simulink model "Week3_Problem3"  (R2020b)
settings: Solver=ode45  StartTime=0.0  StopTime=10.0  RelTol=1e-3
PreLoadFcn:
  | LookupTableVariables.m
PostLoadFcn:
  | posRef=[-10 0 0;-8.5000000389649344 -0.00032057688834367633 0;-7.00000013243916 0.0001046627707353404 0;-5.5000013719066843 0.0019633028915715441 0;-4.0000068200170222 0.0059429239765455251 0;-2.500022456114432 0.012731095719916501 0;-1.000058121729845 0.023015362926791384 0;0.49987153401052709 0.037483222580328462 0;1.9997488741214804 0.05661776191230368 0;3.4995533957878173 0.0807832726616669 0;4.9992537956041394 0.11070949504224792 0;6.4988102169399058 0.14713214905782759 0;7.99817323834591 0.19078661801418004 0;9.4972827923589911 0.24240782912164788 0;10.996067085850811 0.3027301079820538 0;12.494441522418191 0.37248700431913734 0;13.992307627411369 0.45241108632067739 0;15.489552329450575 0.54322828982636229 0;16.986104748171872 0.64482692871996372 0;18.481993555798578 0.75577957443767907 0;19.977281971545665 0.87455822436566311 0;21.472057156443615 0.99963648279861006 0;22.966425539696488 1.1294893996997795 0;24.46050815174387 1.2625932112379594 0;25.954435963048805 1.3974250059040985 0;27.448345227102681 1.5324623399719128 0;28.942364285176254 1.6662786950018476 0;30.43653068335416 1.7984397038989934 0;31.93085365809711 1.9288182087711181 0;33.425345542750946 2.0572458498503861 0;34.920018011779121 2.1835542137146304 0;36.414882023832668 2.3075748302864034 0;37.909947764790829 2.429139170234988 0;39.405224590771311 2.5480786428134428 0;40.900720971109862 2.6642245941628082 0;42.396444431308815 2.7774083061155972 0;43.892403246150053 2.8874369946783749 0;45.38861538488505 2.9939643927789104 0;46.885100476364542 3.096584841736945 0;48.381874979464556 3.1948924196190918 0;49.878951847726285 3.2884810058016432 0;51.37634019890595 3.3769442815837016 0;52.874044984321365 3.4598757359962891 0;54.372066658021069 3.5368686772556726 0;55.870400845812341 3.6075162503092817 0;57.369038014196278 3.671411460922684 0;58.8679627576989 3.7281578592117861 0;60.367140794768574 3.7777688127128712 0;61.866523659152122 3.8207531578250689 0;63.366068909506666 3.8576478218748256 0;64.865740653375155 3.88899000870342 0;66.3655089701928 3.9153171356111991 0;67.865349333770865 3.937166781005621 0;69.365242034387677 3.9550766417191987 0;70.865171600593058 3.9695844989622167 0;72.365126220810183 3.9812281918741537 0;73.865097164799934 3.9905455976371416 0;75.365078205036667 3.9980746171143191 0;76.86506555014661 4.0042226492204165 0;78.365058007335023 4.0089633882717308 0;79.86505400366265 4.0124108908590994 0;81.36505223070516 4.0146952649335228 0;82.8650516827077 4.0159466197411575 0;84.3650516227284 4.0162950653504659 0;85.865051548781452 4.01587071229594 0;87.365051159979728 4.01480367132374 0;88.865050322677291 4.013224053224536 0;90.365049036611751 4.0112619687388946 0;91.865047401046667 4.0090475285205036 0;93.365045580914 4.0067108431425709 0;94.865043772956454 4.0043820231326963 0;96.365042171870044 4.0021911790215441 0;97.865040936446476 4.0002684213906274 0;99.365040171863072 3.9987605666119856 0;100.86503980649982 3.9977214126735334 0;102.36503967169195 3.9970952314177151 0;103.86503964436331 3.9968249528974638 0;105.36503964206052 3.9968535071325086 0;106.86503961643893 3.9971238241271045 0;108.36503954674873 3.997578833881275 0;109.86503943332092 3.9981614663968053 0;111.36503929105332 3.9988146516792265 0;112.86503914289671 3.9994813197370265 0]
  | t= [0 0.099999999999999992 0.20000000000000004 0.3000000000000001 0.40000000000000019 0.50000000000000022 0.60000000000000031 0.7000000000000004 0.80000000000000049 0.90000000000000058 1.0000000000000007 1.1000000000000008 1.2000000000000008 1.3000000000000009 1.400000000000001 1.5000000000000011 1.6000000000000012 1.7000000000000013 1.8000000000000014 1.9000000000000015 2.0000000000000013 2.0999999999999992 2.1999999999999971 2.2999999999999949 2.3999999999999928 2.4999999999999907 2.5999999999999885 2.6999999999999864 2.7999999999999843 2.8999999999999821 2.99999999999998 3.0999999999999779 3.1999999999999758 3.2999999999999736 3.3999999999999715 3.4999999999999694 3.5999999999999672 3.6999999999999651 3.799999999999963 3.8999999999999608 3.9999999999999587 4.099999999999957 4.1999999999999549 4.2999999999999527 4.3999999999999506 4.4999999999999485 4.5999999999999464 4.6999999999999442 4.7999999999999421 4.89999999999994 4.9999999999999378 5.0999999999999357 5.1999999999999336 5.2999999999999314 5.3999999999999293 5.4999999999999272 5.599999999999925 5.6999999999999229 5.7999999999999208 5.8999999999999186 5.9999999999999165 6.0999999999999144 6.1999999999999122 6.29999999999991 6.399999999999908 6.4999999999999059 6.5999999999999037 6.6999999999999016 6.7999999999998995 6.8999999999998973 6.9999999999998952 7.0999999999998931 7.1999999999998909 7.2999999999998888 7.3999999999998867 7.4999999999998845 7.5999999999998824 7.69999999999988 7.7999999999998781 7.899999999999876 7.9999999999998739 8.0999999999998717 8.19999999999987]
  | yawRef = [-0.017734585131802181 -0.0023783867480744541 0.039241603596663142 0.10712538590241065 0.20127296016916807 0.32168432639693528 0.46835948458571258 0.64129843473549952 0.82243120441432782 1.0284466171618847 1.2625895772261897 1.5248600846072435 1.8152581393050453 2.133783741319597 2.4804368906508958 2.8552175872989438 3.2581258312637407 3.6852031921171342 4.0725918737692446 4.4015950546183911 4.6722127346645754 4.8844449139077941 5.0382915923480533 5.1337527699853531 5.1708284468196917 5.1495186228510716 5.0867585477276682 5.02163347038271 4.95006090740082 4.872040858781995 4.787573324526238 4.6966583046335471 4.5992957991039214 4.4954858079373627 4.3852283311338685 4.268523368693443 4.1421046794896679 4.00026229516887 3.8429080694151376 3.6700420022284757 3.4816640936088827 3.2777743435563571 3.058372752070901 2.823459319152513 2.5730340448011941 2.3070969290169434 2.0288148473761831 1.7653020474819436 1.522336655896058 1.2999186726185261 1.0980480976493481 0.91672493098852348 0.75594917263605244 0.61572082259193561 0.49603988085617257 0.39690634742876296 0.3183202223097073 0.26028150549900531 0.20743891230476702 0.155555799189824 0.10864254782766856 0.066699158218300636 0.029725630361720226 -0.0022780357420727169 -0.0293118400930781 -0.051375782691295953 -0.068469863536726308 -0.080594082629369151 -0.087748439969224434 -0.0899329355562922 -0.087147569390572471 -0.079392341472065239 -0.066667251800770516 -0.04830659623807302 -0.031442242528749914 -0.016757802096312908 -0.004253274940762026 0.0060713389379027606 0.014216039539681403 0.020180826864573963 0.023965700912580403 0.025570661683700712 0.024995709177934915]
model workspace (MAT data in the model file):
  mpc1 = mpc
  mpc1.Ts = 0.1
  mpc1.PredictionHorizon = 10
  mpc1.ControlHorizon = 3
  mpc1.Model.Plant = ss
  mpc1.Model.Plant.InputName_ = "Steering angle"
  mpc1.Model.Plant.InputUnit_ = "rad"
  mpc1.Model.Plant.InputGroup_.Manipulated = 1
  mpc1.Model.Plant.OutputName_ = ["Lateral position"; "Yaw angle"]
  mpc1.Model.Plant.OutputUnit_ = ["m"; "rad"]
  mpc1.Model.Plant.OutputGroup_.Measured = [1 2]
  mpc1.Model.Plant.IOSize_ = [2 1]
  mpc1.Model.Plant.Data_ = ltipack.ssdata
  mpc1.Model.Plant.Data_.StateName = ["Plant(1)"; "Plant(2)"; "Plant(3)"; "Plant(4)"]
  mpc1.Model.Plant.Data_.a = [0.590295220137  0  -0.749548819532  0; 0.00501866857034  1  0.0760340469864  0; 0.0836937369247  0  0.543093723808  0; 0.0815953844705  1.5  0.0178017333486  1]
  mpc1.Model.Plant.Data_.b = [1.18987189092; 0.0707419750471; 1.3270514387; 0.114007098227]
  mpc1.Model.Plant.Data_.c = [0  0  0  1; 0  1  0  0]
  mpc1.Model.Plant.Data_.d = [0; 0]
  mpc1.Model.Plant.Data_.Delay.Input = 0
  mpc1.Model.Plant.Data_.Delay.Output = [0; 0]
  mpc1.Model.Plant.Data_.Delay.Internal = []
  mpc1.Model.Plant.Data_.Ts = 0.1
  mpc1.Model.Disturbance = []
  mpc1.Model.Noise = []
  mpc1.Model.Nominal.X = [0; 0; 0; 0]
  mpc1.Model.Nominal.DX = [0; 0; 0; 0]
  mpc1.Model.Nominal.U = 0
  mpc1.Model.Nominal.Y = [0; 0]
  mpc1.ManipulatedVariables.Min = -0.523598775598
  mpc1.ManipulatedVariables.Max = 0.523598775598
  mpc1.ManipulatedVariables.MinECR = 0
  mpc1.ManipulatedVariables.MaxECR = 0
  mpc1.ManipulatedVariables.RateMin = -0.261799387799
  mpc1.ManipulatedVariables.RateMax = 0.261799387799
  mpc1.ManipulatedVariables.RateMinECR = 0
  mpc1.ManipulatedVariables.RateMaxECR = 0
  mpc1.ManipulatedVariables.Target = 'nominal'
  mpc1.ManipulatedVariables.Name = 'Steering angle'
  mpc1.ManipulatedVariables.Units = 'rad'
  mpc1.ManipulatedVariables.ScaleFactor = 1
  mpc1.OutputVariables(1).Min = -2
  mpc1.OutputVariables(1).Max = 6
  mpc1.OutputVariables(1).MinECR = 1
  mpc1.OutputVariables(1).MaxECR = 1
  mpc1.OutputVariables(1).Name = 'Lateral position'
  mpc1.OutputVariables(1).Units = 'm'
  mpc1.OutputVariables(1).ScaleFactor = 1
  mpc1.OutputVariables(2).Min = -0.2
  mpc1.OutputVariables(2).Max = 0.2
  mpc1.OutputVariables(2).MinECR = 1
  mpc1.OutputVariables(2).MaxECR = 1
  mpc1.OutputVariables(2).Name = 'Yaw angle'
  mpc1.OutputVariables(2).Units = 'rad'
  mpc1.OutputVariables(2).ScaleFactor = 1
  mpc1.Weights.ManipulatedVariables = 0
  mpc1.Weights.ManipulatedVariablesRate = 0.0353454681959
  mpc1.Weights.OutputVariables = [2.82921701435 0.282921701435]
  mpc1.Weights.ECR = 100000
  mpc1.Optimizer.Algorithm = 'active-set'
  mpc1.Optimizer.ActiveSetOptions.MaxIterations = 'default'
  mpc1.Optimizer.ActiveSetOptions.ConstraintTolerance = 1e-06
  mpc1.Optimizer.ActiveSetOptions.UseWarmStart = 1
  mpc1.Optimizer.InteriorPointOptions.MaxIterations = 50
  mpc1.Optimizer.InteriorPointOptions.ConstraintTolerance = 1e-06
  mpc1.Optimizer.InteriorPointOptions.OptimalityTolerance = 1e-06
  mpc1.Optimizer.InteriorPointOptions.ComplementarityTolerance = 1e-08
  mpc1.Optimizer.InteriorPointOptions.StepTolerance = 1e-08
  mpc1.Optimizer.MinOutputECR = 0
  mpc1.Optimizer.UseSuboptimalSolution = 0
  mpc1.Optimizer.CustomSolver = 0
  mpc1.Optimizer.CustomSolverCodeGen = 0
  mpc1.History = [2018 8 28 11 8 30.674]
  mpc1.MPCData = mpcdata
  mpc1.MPCData.IsDirty = 1
  mpc1.MPCData.Ts = 0.1
  mpc1.MPCData.p = 10
  mpc1.MPCData.m = 3
  mpc1.MPCData.UseActiveSetSolver = 1
  mpc1.MPCData.UseSuboptimalSolution = 0
  mpc1.MPCData.CustomSolver = 0
  mpc1.MPCData.CustomSolverCodeGen = 0
  mpc1.MPCData.IsCustomEstimation = 0
  mpc1.MPCData.Uscale = 1
  mpc1.MPCData.Yscale = [1; 1]
  mpc1.MPCData.mvindex = 1
  mpc1.MPCData.myindex = [1; 2]
  mpc1.IsEmpty = 0
  mpc1.OldOVIntegrator = {[]; []}
  mpc1.Version = '6.1'
  posRef = [-10 -8.50000003896 -7.00000013244 -5.50000137191 -4.00000682002 -2.50002245611 -1.00005812173 0.499871534011 1.99974887412 3.49955339579 4.9992537956 6.49881021694 ... (249 elements, 83x3)]
  t = [0 0.1 0.2 0.3 0.4 0.5 0.6 0.7 0.8 0.9 1 1.1 1.2 1.3 1.4 1.5 1.6 1.7 1.8 1.9 2 2.1 2.2 2.3 2.4 2.5 2.6 2.7 2.8 2.9 3 3.1 3.2 3.3 3.4 3.5 3.6 3.7 3.8 3.9 4 4.1 4.2 4.3 4.4 4.5 4.6 4.7 4.8 4.9 5 5.1 5.2 5.3 5.4 5.5 5.6 5.7 5.8 5.9 6 6.1 6.2 6.3 6.4 6.5 6.6 6.7 6.8 6.9 7 7.1 7.2 7.3 7.4 7.5 7.6 7.7 7.8 7.9 8 8.1 8.2]
  yawRef = [-0.0177345851318 -0.00237838674807 0.0392416035967 0.107125385902 0.201272960169 0.321684326397 0.468359484586 0.641298434735 0.822431204414 1.02844661716 1.26258957723 1.52486008461 1.81525813931 2.13378374132 2.48043689065 2.8552175873 3.25812583126 3.68520319212 4.07259187377 4.40159505462 4.67221273466 4.88444491391 5.03829159235 5.13375276999 5.17082844682 5.14951862285 5.08675854773 5.02163347038 4.9500609074 4.87204085878 4.78757332453 4.69665830463 4.5992957991 4.49548580794 4.38522833113 4.26852336869 4.14210467949 4.00026229517 3.84290806942 3.67004200223 3.48166409361 3.27777434356 3.05837275207 2.82345931915 2.5730340448 2.30709692902 2.02881484738 1.76530204748 1.5223366559 1.29991867262 1.09804809765 0.916724930989 0.755949172636 0.615720822592 0.496039880856 0.396906347429 0.31832022231 0.260281505499 0.207438912305 0.15555579919 0.108642547828 0.0666991582183 0.0297256303617 -0.00227803574207 -0.0293118400931 -0.0513757826913 -0.0684698635367 -0.0805940826294 -0.0877484399692 -0.0899329355563 -0.0871475693906 -0.0793923414721 -0.0666672518008 -0.0483065962381 -0.0314422425287 -0.0167578020963 -0.00425327494076 0.0060713389379 0.0142160395397 0.0201808268646 0.0239657009126 0.0255706616837 0.0249957091779]
values from neighbouring files (symbols this model uses):
  desiredLong = [20 24 30]    [LookupTableVariables.m]
  givenLong = [ 10 12 15]    [LookupTableVariables.m]
undefined symbols (not defined in the file or in its folder): sigbuilder_block
libraries: mpclib x1
CloseFcn:
  | clearvars
settings Model: OrderedModelArguments=off  Creator=hp  LastModifiedBy=hp

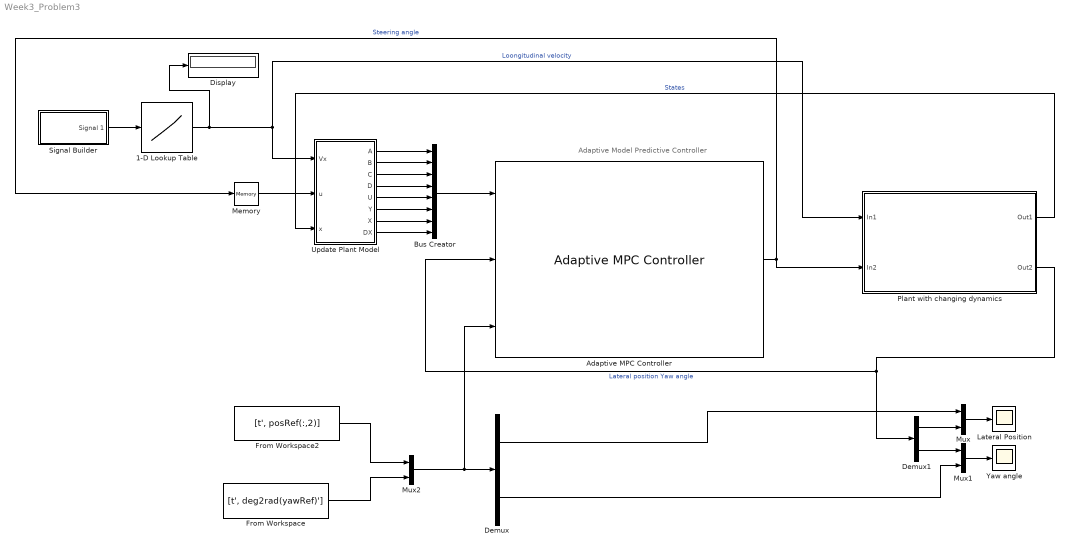
== system Week3_Problem3 ==
  note: Adaptive Model Predictive Controller
  1-D Lookup Table : Lookup_n-D  NumberOfTableDimensions=1  BreakpointsForDimension1=givenLong  Table=desiredLong  InternalRulePriority=Speed  RndMeth=Simplest  InputSameDT=on
  Adaptive MPC Controller : mpclib/Adaptive MPC Controller  SCDEnableBlockLinearizationSpecification=on  mpcobj=mpc1  enable_value=0  updateMPCinCallerWorkspace=on  md_inport=off  mv_inport=off  uref_inport=off  return_cost=off  return_mvseq=off  return_qpstatus=off  return_xseq=off  return_state=off  return_ovseq=off  state_inport=off  isltv_plant=off  umin_inport=off  umax_inport=off  ymin_inport=off  ymax_inport=off  cc_inport=off  ywt_inport=off  uwt_inport=off  duwt_inport=off  rhoeps_inport=off  pm_inport=off  MaximumP=10  HorizonChoice=FixedHorizon  BlockDataType=double  SampleTimeInherited=off  switch_inport=off  mask(Adaptive MPC){}
      mask Display: image('C:\Users\hp\Desktop\MPC.PNG'); % Use "Edit Image" on toolstrip to change.
  Bus Creator : BusCreator  Inputs=8
  Demux : Demux  Outputs=2
  Demux1 : Demux  Outputs=2
  Display : Display
  From Workspace : FromWorkspace  VariableName=[t', deg2rad(yawRef)']  SampleTime=0.1
  From Workspace2 : FromWorkspace  VariableName=[t', posRef(:,2)]  SampleTime=0.1
  Lateral Position : Scope
  Memory : Memory
  Mux : Mux  Inputs=2
  Mux1 : Mux  Inputs=2
  Mux2 : Mux  Inputs=2
  Plant with changing dynamics : Subsystem
      mask Display: image('C:\Users\hp\Desktop\Q3.PNG'); % Use "Edit Image" on toolstrip to change.
  Signal Builder : Subsystem  Tag=STV Subsys  LoadFcn=sigbuilder_block('load');  StartFcn=sigbuilder_block('start');  StopFcn=sigbuilder_block('stop');  ClipboardFcn=sigbuilder_block('clipboard');  mask(Sigbuilder block){tuvar=[0:10]}
      mask help: Simulink:masks:SigbuilderBlock_MD
      mask init:
      | if ~strcmp(get_param(bdroot(gcbh),'SimulationStatus'),'stopped') tuvar = sigbuilder_block('maskInit'); end
      settings: CopyFcn=sigbuilder_block('copy');  DeleteFcn=sigbuilder_block('delete');  ModelCloseFcn=sigbuilder_block('modelClose');  PreSaveFcn=sigbuilder_block('preSave');  PauseFcn=sigbuilder_block('pause');  ContinueFcn=sigbuilder_block('continue');  NameChangeFcn=sigbuilder_block('namechange');  OpenFcn=sigbuilder_block('open',[437.6 153 550.4 359.25 ]);  CloseFcn=sigbuilder_block('close');
      mask Display: plot(0, 0, 100, 100,[2, 2, 32, 32, 2], [68, 8, 8, 68, 68],[32, 2], [38, 38], [32, 19, 2],[53, 60, 44], [32, 17, 17, 2],[16, 16, 31, 31]);txt = getActiveGroup(gcbh);text(2, 100, txt,'verticalAlignment', 'top');
  Update Plant Model : MATLAB Function  TreatAsAtomicUnit=on
  Yaw angle : Scope
  wires:
  Update Plant Model/3(C) -> Bus Creator/3
  Mux/1 -> Lateral Position/1
  From Workspace/1 -> Mux2/2
  Adaptive MPC Controller/1 -> Memory/1, Plant with changing dynamics/2(In2)  "Steering angle"
  Mux1/1 -> Yaw angle/1
  Plant with changing dynamics/1(Out1) -> Update Plant Model/3(x)  "States"
  Demux/2 -> Mux1/2
  Demux/1 -> Mux/1
  Demux1/2 -> Mux1/1
  Plant with changing dynamics/2(Out2) -> Demux1/1, Adaptive MPC Controller/2  "Lateral position Yaw angle"
  From Workspace2/1 -> Mux2/1
  Memory/1 -> Update Plant Model/2(u)
  Mux2/1 -> Adaptive MPC Controller/3, Demux/1
  Demux1/1 -> Mux/2
  Update Plant Model/5(U) -> Bus Creator/5
  Update Plant Model/1(A) -> Bus Creator/1
  Update Plant Model/6(Y) -> Bus Creator/6
  Bus Creator/1 -> Adaptive MPC Controller/1
  Update Plant Model/2(B) -> Bus Creator/2
  Update Plant Model/8(DX) -> Bus Creator/8
  Update Plant Model/4(D) -> Bus Creator/4
  1-D Lookup Table/1 -> Display/1, Update Plant Model/1(Vx), Plant with changing dynamics/1(In1)  "Loongitudinal velocity"
  Update Plant Model/7(X) -> Bus Creator/7
  Signal Builder/1(Signal 1) -> 1-D Lookup Table/1

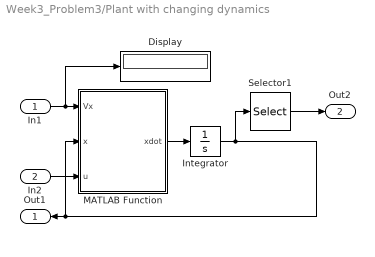
== system Week3_Problem3/Plant with changing dynamics ==
  In1 : Inport
  In2 : Inport  Port=2
  Display : Display
  Integrator : Integrator
  MATLAB Function : MATLAB Function  TreatAsAtomicUnit=on
  Selector1 : Selector  InputPortWidth=4  IndexOptions=Index vector (dialog)  Indices=[4 2]  OutputSizes=1
  Out1 : Outport  VectorParamsAs1DForOutWhenUnconnected=off
  Out2 : Outport  Port=2  VectorParamsAs1DForOutWhenUnconnected=off
  wires:
  In2/1 -> MATLAB Function/3(u)
  In1/1 -> Display/1, MATLAB Function/1(Vx)
  Integrator/1 -> Selector1/1, MATLAB Function/2(x), Out1/1
  MATLAB Function/1(xdot) -> Integrator/1
  Selector1/1 -> Out2/1

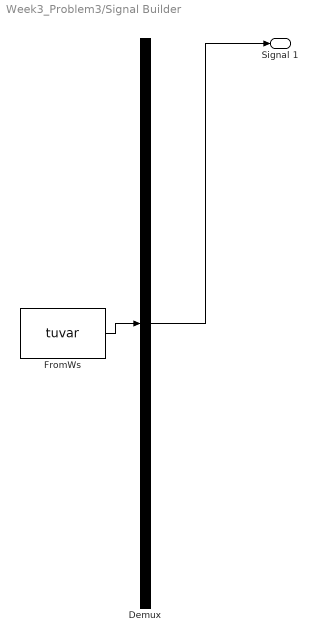
== system Week3_Problem3/Signal Builder ==
  Demux : Demux  Tag=STV Demux  Outputs=1
      settings: DisplayOption=none
  FromWs : FromWorkspace  Tag=STV FromWs  VariableName=tuvar
      SigBuilderData=|
      | common.afterFinalStr = 'Extrapolate'
      | common.sampleTime = 0
      | dataSet.timeRange = [0 10]
      | dataSet.name = 'Group 1'
      | sbobj.Groups.Name = 'Group 1'
      | sbobj.Groups.Signals.Name = 'Signal 1'
      | sbobj.Groups.Signals.XData = [0 4 4 5.98 10]
      | sbobj.Groups.Signals.YData = [10 10 12 12 12]
  Signal 1 : Outport  Tag=STV Outport
  wires:
  Demux/1 -> Signal 1/1
  FromWs/1 -> Demux/1

== matlab function Week3_Problem3/Plant with changing dynamics/MATLAB Function ==
  data: Vx input; x input size=[4,1]; u input; xdot output size=[4,1]
function xdot = fcn(Vx,x,u)

% Model parameters
m = 1575;
Iz = 2875;
lf = 1.2;
lr = 1.6;
Cf = 19000;
Cr = 33000;

% Continuous-time model
A = [-(2*Cf+2*Cr)/m/Vx, 0, -Vx-(2*Cf*lf-2*Cr*lr)/m/Vx, 0;
     0, 0, 1, 0;
     -(2*Cf*lf-2*Cr*lr)/Iz/Vx, 0, -(2*Cf*lf^2+2*Cr*lr^2)/Iz/Vx, 0;
     1, Vx, 0, 0];
B = [2*Cf/m 0 2*Cf*lf/Iz 0]';   
C = [0 0 0 1; 0 1 0 0];
D = zeros(2,1);
xdot = A*x + B*u;
%y = C*x + D*u;

== matlab function Week3_Problem3/Update Plant Model ==
  data: Vx input; u input; A output size=[4,4]; x input size=[4,1]; B output size=[4,1]; C output size=[2,4]; D output size=[2,1]; U output; Y output size=[2,1]; X output size=[4,1]; DX output size=[4,1]
function [A,B,C,D,U,Y,X,DX] = fcn(Vx,u,x)
% Sample time
Ts = 0.1;

% Model parameters
m = 1575;
Iz = 2875;
lf = 1.2;
lr = 1.6;
Cf = 19000;
Cr = 33000;

% Continuous-time model
Ac = [-(2*Cf+2*Cr)/m/Vx, 0, -Vx-(2*Cf*lf-2*Cr*lr)/m/Vx, 0;
     0, 0, 1, 0;
     -(2*Cf*lf-2*Cr*lr)/Iz/Vx, 0, -(2*Cf*lf^2+2*Cr*lr^2)/Iz/Vx, 0;
     1, Vx, 0, 0];
Bc = [2*Cf/m 0 2*Cf*lf/Iz 0]';   
Cc = [0 0 0 1; 0 1 0 0];
Dc = zeros(2,1);

% Generate discrete-time model
nx = size(Ac,1);
nu = size(Bc,2);
M = expm([[Ac Bc]*Ts; zeros(nu,nx+nu)]);
A = M(1:nx,1:nx);
B = M(1:nx,nx+1:nx+nu);
C = Cc;
D = Dc;

% Nominal conditions for discrete-time plant
X = x;
U = u;
Y = C*x + D*u;
DX = A*x+B*u-x;
